simulink model "auv_sonar_payload_top"  (R2026a)
settings: Solver=FixedStepDiscrete  StopTime=t_mission_end  FixedStep=Ts_ping
PreLoadFcn:
  | % Self-healing path configuration for AUV Sonar Simulink Suite
  | m_file = get_param(bdroot, 'FileName');
  | if ~isempty(m_file)
  |     m_dir = fileparts(m_file);
  |     addpath(m_dir);
  |     addpath(fullfile(m_dir, '..'));
  | else
  |     if exist(fullfile(pwd, 'matlab', 'simulink'), 'dir')
  |         addpath(fullfile(pwd, 'matlab', 'simulink'));
  |         addpath(fullfile(pwd, 'matlab'));
  |     end
  | end
  | if exist('init_sonar_simulink', 'file') == 2
  |     init_sonar_simulink;
  | end
InitFcn:
  | % Self-healing path configuration for AUV Sonar Simulink Suite
  | m_file = get_param(bdroot, 'FileName');
  | if ~isempty(m_file)
  |     m_dir = fileparts(m_file);
  |     addpath(m_dir);
  |     addpath(fullfile(m_dir, '..'));
  | else
  |     if exist(fullfile(pwd, 'matlab', 'simulink'), 'dir')
  |         addpath(fullfile(pwd, 'matlab', 'simulink'));
  |         addpath(fullfile(pwd, 'matlab'));
  |     end
  | end
  | if exist('init_sonar_simulink', 'file') == 2
  |     init_sonar_simulink;
  | end
undefined symbols (not defined in the file or in its folder): Ts_ping
settings Model: Creator=harsh  LastModifiedBy=harsh

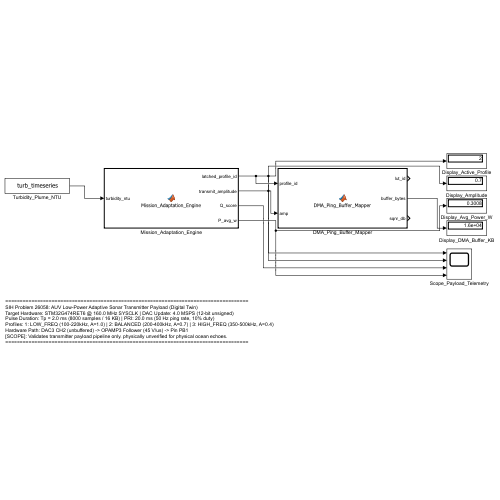
[thumbnail: Simulink's stored preview of the top-level diagram]
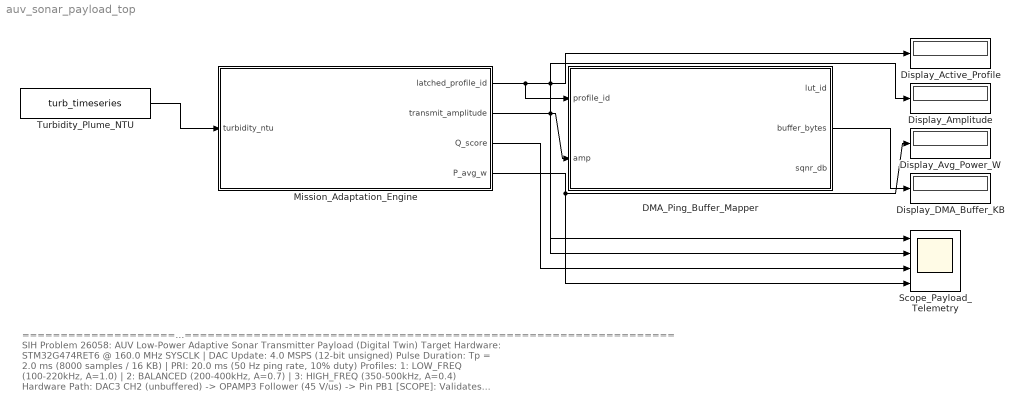
== system auv_sonar_payload_top ==
  note: ====================================================================================
      | SIH Problem 26058: AUV Low-Power Adaptive Sonar Transmitter Payload (Digital Twin)
      | Target Hardware: STM32G474RET6 @ 160.0 MHz SYSCLK | DAC Update: 4.0 MSPS (12-bit unsigned)
      | Pulse Duration: Tp = 2.0 ms (8000 samples / 16 KB) | PRI: 20.0 ms (50 Hz ping rate, 10% duty)
      | Profiles: 1: LOW_FREQ (100-220kHz, A=1.0) | 2: BALANCED (200-400kHz, A=0.7) | 3: HIGH_FREQ (350-500kHz, A=0.4)
      | Hardware Path: DAC3 CH2 (unbuffered) -> OPAMP3 Follower (45 V/us) -> Pin PB1
      | [SCOPE]: Validates transmitter payload pipeline only. physically unverified for physical ocean echoes.
      | ====================================================================================
  DMA_Ping_Buffer_Mapper : MATLAB Function  TreatAsAtomicUnit=on
  Display_Active_Profile : Display
  Display_Amplitude : Display
  Display_Avg_Power_W : Display
  Display_DMA_Buffer_KB : Display
  Mission_Adaptation_Engine : MATLAB Function  TreatAsAtomicUnit=on
  Scope_Payload_Telemetry : Scope  NumInputPorts=4
      settings: ActiveDisplayYMinimum=-1.5745756601935068  ActiveDisplayYMaximum=4.139018406829857
  Turbidity_Plume_NTU : FromWorkspace  VariableName=turb_timeseries  SampleTime=Ts_ping  OutputAfterFinalValue=Holding final value
  wires:
  Turbidity_Plume_NTU/1 -> Mission_Adaptation_Engine/1(turbidity_ntu)
  Mission_Adaptation_Engine/1(latched_profile_id) -> Display_Active_Profile/1, Scope_Payload_Telemetry/1, DMA_Ping_Buffer_Mapper/1(profile_id)
  Mission_Adaptation_Engine/2(transmit_amplitude) -> DMA_Ping_Buffer_Mapper/2(amp), Display_Amplitude/1, Scope_Payload_Telemetry/2
  Mission_Adaptation_Engine/3(Q_score) -> Scope_Payload_Telemetry/3
  Mission_Adaptation_Engine/4(P_avg_w) -> Display_Avg_Power_W/1, Scope_Payload_Telemetry/4
  DMA_Ping_Buffer_Mapper/2(buffer_bytes) -> Display_DMA_Buffer_KB/1

== matlab function auv_sonar_payload_top/DMA_Ping_Buffer_Mapper ==
  data: profile_id input; lut_id output; amp input; buffer_bytes output; sqnr_db output
function [lut_id, buffer_bytes, sqnr_db] = DMA_Ping_Buffer_Mapper(profile_id, amp)
lut_id = double(profile_id);
buffer_bytes = 16000.0; % 8000 samples * 2 bytes (uint16)
sqnr_db = 69.5;
if profile_id == 1
    sqnr_db = 70.8;
elseif profile_id == 3
    sqnr_db = 68.2;
end
end

== matlab function auv_sonar_payload_top/Mission_Adaptation_Engine ==
  data: turbidity_ntu input; latched_profile_id output; transmit_amplitude output; Q_score output; P_avg_w output
function [latched_profile_id, transmit_amplitude, Q_score, P_avg_w] = ...
    Mission_Adaptation_Engine(turbidity_ntu)
coder.extrinsic('sim_bridge_channel', 'sim_bridge_controller', 'sim_bridge_power');
latched_profile_id = 2.0;
transmit_amplitude = 0.70;
Q_score = 0.50;
P_avg_w = 0.30;
[Q_score, ~, ~, ~, ~, ~] = sim_bridge_channel(turbidity_ntu, 50.0, 20.0, 35.0, 55.0, 50.0, 1.0);
[latched_profile_id, ~, ~, ~, transmit_amplitude] = sim_bridge_controller(Q_score);
[P_avg_w, ~, ~, ~] = sim_bridge_power(transmit_amplitude, 0.002);
end
